simulink model "Separator1"  (R2018b)
settings: Solver=VariableStepAuto  StartTime=0.0  StopTime=10.0  RelTol=1e-3
settings Model: Creator=smf52  LastModifiedBy=art58

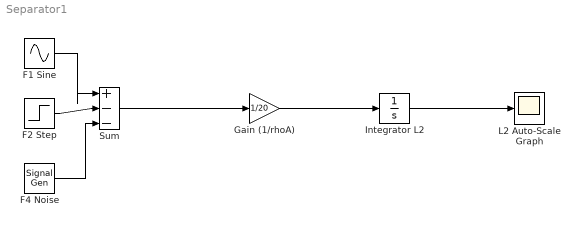
== system Separator1 ==
  "F1 Sine " : Sin  SampleTime=0
  F2 Step : Step  SampleTime=0
  F4 Noise : SignalGenerator  Units=rad/sec
  Gain (1/rhoA) : Gain  Gain=1/20
  "Integrator L2 " : Integrator
  L2 Auto-Scale Graph : Scope
  Sum : Sum  Inputs=|+--
  wires:
  Sum/1 -> Gain (1/rhoA)/1
  Gain (1/rhoA)/1 -> "Integrator L2 "/1
  "Integrator L2 "/1 -> L2 Auto-Scale Graph/1
  "F1 Sine "/1 -> Sum/1
  F2 Step/1 -> Sum/2
  F4 Noise/1 -> Sum/3
